simulink model "bai1_2input_PD_fuzzy"  (R2017b)
settings: Solver=ode5  StartTime=0.0  StopTime=60  FixedStep=0.1  RelTol=1e-3
undefined symbols (not defined in the file or in its folder): sigbuilder_block
libraries: fuzblock x1
settings Model: Creator=phamt  LastModifiedBy=phamt

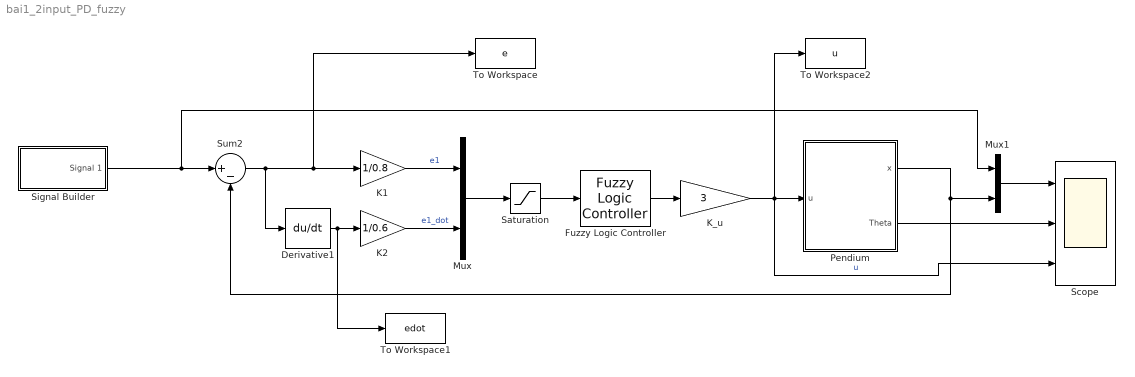
== system bai1_2input_PD_fuzzy ==
  Derivative1 : Derivative
  Fuzzy Logic Controller : fuzblock/Fuzzy Logic  Controller  FIS='bai1_PD_FIS.fis'  OutputSampleNumber=101  DataType=double  FuzzifiedInputs=off  RuleFiringStrengths=off  RuleOutputs=off  AggregatedOutputs=off  SimulateUsing=Interpreted execution
  K1 : Gain  Gain=1/0.8
  K2 : Gain  Gain=1/0.6
  K_u : Gain  Gain=3
  Mux : Mux  Inputs=2
  Mux1 : Mux  Inputs=2
  Pendium : Subsystem  mask{H=0.5, m=2, l=0.6, g=9.81, x0=0.2, xdot0=0.1, theta0=pi/18, thetadot0=0}
      mask prompts: H "M"
  Saturation : Saturate  UpperLimit=1  LowerLimit=-1
  Scope : Scope  NumInputPorts=3
  Signal Builder : Subsystem  Tag=STV Subsys  LoadFcn=sigbuilder_block('load',[0 36 960 449.5 ]);  StartFcn=sigbuilder_block('start');  StopFcn=sigbuilder_block('stop');  ClipboardFcn=sigbuilder_block('clipboard');  mask(Sigbuilder block){tuvar=[0:10]}
      mask help: Simulink:masks:SigbuilderBlock_MD
      mask init:
      | if ~strcmp(get_param(bdroot(gcbh),'SimulationStatus'),'stopped') tuvar = sigbuilder_block('maskInit'); end
      settings: CopyFcn=sigbuilder_block('copy');  DeleteFcn=sigbuilder_block('delete');  ModelCloseFcn=sigbuilder_block('modelClose');  PreSaveFcn=sigbuilder_block('preSave');  PauseFcn=sigbuilder_block('pause');  ContinueFcn=sigbuilder_block('continue');  NameChangeFcn=sigbuilder_block('namechange');  OpenFcn=sigbuilder_block('open',[437.6 199.2 550.4 400 ]);  CloseFcn=sigbuilder_block('close');
      mask Display: plot(0, 0, 100, 100,[2, 2, 32, 32, 2], [68, 8, 8, 68, 68],[32, 2], [38, 38], [32, 19, 2],[53, 60, 44], [32, 17, 17, 2],[16, 16, 31, 31]);txt = getActiveGroup(gcbh);text(2, 100, txt,'verticalAlignment', 'top');
  Sum2 : Sum  Inputs=|+-
  To Workspace : ToWorkspace  VariableName=e  SampleTime=-1
  To Workspace1 : ToWorkspace  VariableName=edot  SampleTime=-1
  To Workspace2 : ToWorkspace  VariableName=u  SampleTime=-1
  wires:
  Pendium/1(x) -> Mux1/2, Sum2/2
  Signal Builder/1(Signal 1) -> Mux1/1, Sum2/1
  K_u/1 -> To Workspace2/1, Scope/3, Pendium/1(u)  "u"
  Saturation/1 -> Fuzzy Logic Controller/1
  Fuzzy Logic Controller/1 -> K_u/1
  Mux1/1 -> Scope/1
  Pendium/2(Theta) -> Scope/2
  K1/1 -> Mux/1  "e1"
  Sum2/1 -> Derivative1/1, To Workspace/1, K1/1
  Mux/1 -> Saturation/1
  Derivative1/1 -> To Workspace1/1, K2/1
  K2/1 -> Mux/2  "e1_dot"

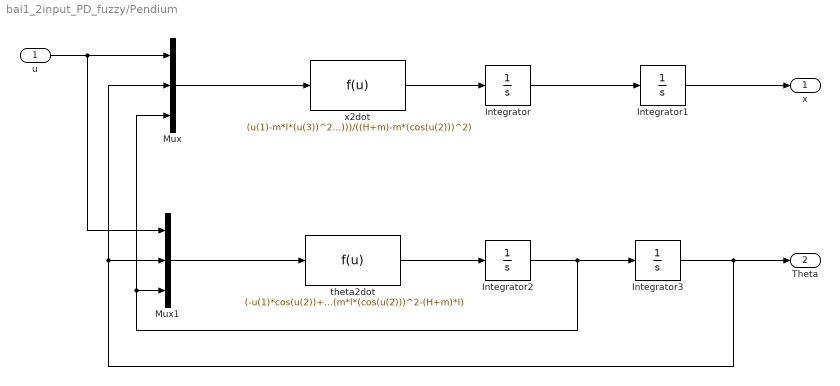
== system bai1_2input_PD_fuzzy/Pendium ==
  u : Inport
  Integrator : Integrator  InitialCondition=xdot0
  Integrator1 : Integrator  InitialCondition=x0
  Integrator2 : Integrator  InitialCondition=thetadot0
  Integrator3 : Integrator  InitialCondition=theta0
  Mux : Mux  Inputs=3
  Mux1 : Mux  Inputs=3
  theta2dot : Fcn  Expr=(-u(1)*cos(u(2))+m*g*(u(3))^2*sin(u(2))*cos(u(2))+(H+m)*(g*sin(u(2))))/(m*l*(cos(u(2)))^2-(H+m)*l)
  x2dot : Fcn  Expr=(u(1)-m*l*(u(3))^2*sin(u(2))-m*g*sin(u(2))*cos(u(2)))/((H+m)-m*(cos(u(2)))^2)
  x : Outport
  Theta : Outport  Port=2
  wires:
  u/1 -> Mux1/1, Mux/1
  Mux/1 -> x2dot/1
  x2dot/1 -> Integrator/1
  Integrator/1 -> Integrator1/1
  Mux1/1 -> theta2dot/1
  Integrator2/1 -> Mux/3, Mux1/3, Integrator3/1
  theta2dot/1 -> Integrator2/1
  Integrator1/1 -> x/1
  Integrator3/1 -> Mux/2, Mux1/2, Theta/1

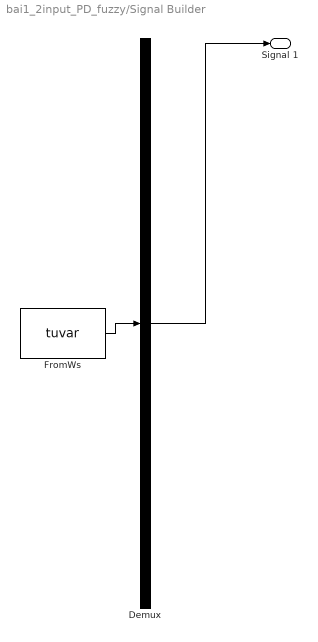
== system bai1_2input_PD_fuzzy/Signal Builder ==
  Demux : Demux  Tag=STV Demux  Outputs=1
  FromWs : FromWorkspace  Tag=STV FromWs  VariableName=tuvar  SampleTime=0
      SigBuilderData=|
      | common.afterFinalStr = 'Extrapolate'
      | common.sampleTime = 0
      | dataSet.timeRange = [0 60]
      | dataSet.name = 'Group 1'
      | sbobj.Groups.Name = 'Group 1'
      | sbobj.Groups.Signals.Name = 'Signal 1'
      | sbobj.Groups.Signals.XData = [0 10 10 20 20 30 30 40 40 50 50 60]
      | sbobj.Groups.Signals.YData = [0.45 0.45 0.2 0.2 0.8 0.8 0.55 0.55 0.1 0.1 0.65 0.65]
      | sbobj.Groups.TimeRange = [0 60]
  Signal 1 : Outport  Tag=STV Outport
  wires:
  Demux/1 -> Signal 1/1
  FromWs/1 -> Demux/1
